simulink model "quadcopter_hover"  (R2022b)
settings: Solver=FixedStepDiscrete  StartTime=0.0  StopTime=40  FixedStep=0.0025  RelTol=1e-3
undefined symbols (not defined in the file or in its folder): f
libraries: instrumentlib x2
settings Model: Creator=HP  LastModifiedBy=HP

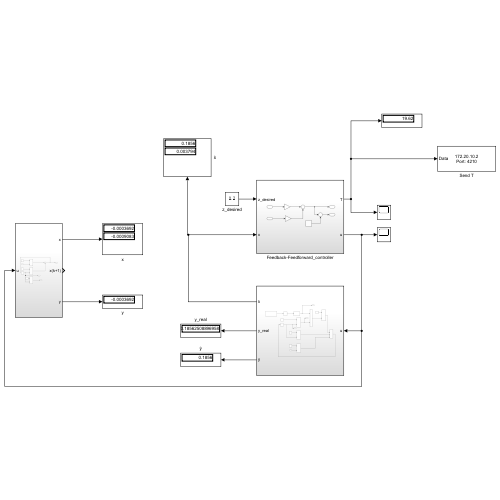
[thumbnail: Simulink's stored preview of the top-level diagram]
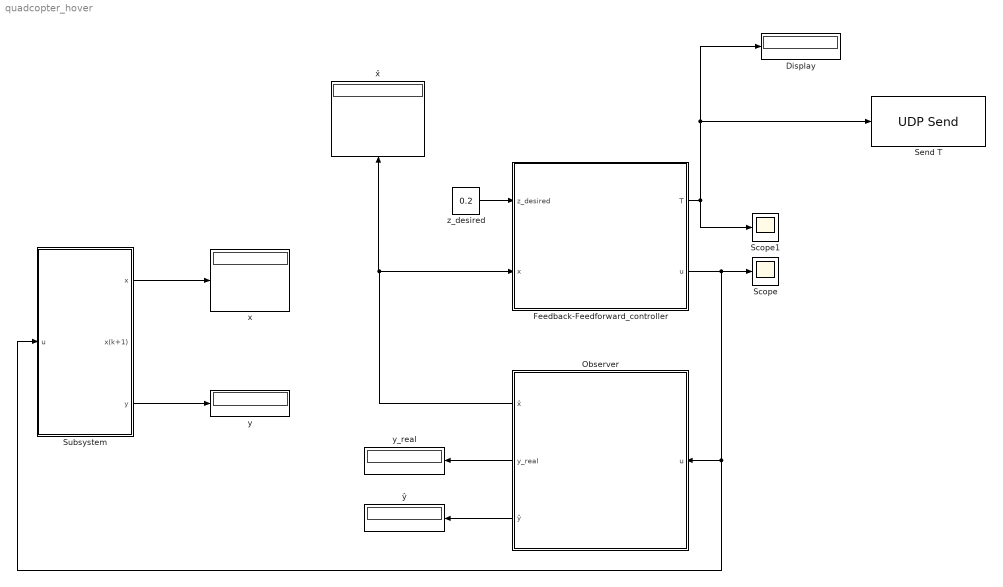
== system quadcopter_hover ==
  Display : Display
  Feedback-Feedforward_controller : Subsystem
  Observer : Subsystem
  Scope : Scope
  Scope1 : Scope
  Send T : instrumentlib/UDP Send  Host=172.20.10.2  Port=4210  LocalAddress=0.0.0.0  LocalPort=4211  EnablePortSharing=off  OutputDatagramPacketSize=512  ByteOrder=big-endian  EnableBlockingMode=on  SimulateUsing=Interpreted execution
  Subsystem : Subsystem
  x : Display
  x̂ : Display
  y : Display
  y_real : Display
  z_desired : Constant  Value=0.2
  ŷ : Display
  wires:
  Feedback-Feedforward_controller/2(u) -> Subsystem/1(u), Observer/1(u), Scope/1
  z_desired/1 -> Feedback-Feedforward_controller/1(z_desired)
  Subsystem/1(x) -> x/1
  Subsystem/3(y) -> y/1
  Observer/1(x̂) -> Feedback-Feedforward_controller/2(x), x̂/1
  Observer/2(y_real) -> y_real/1
  Observer/3(ŷ) -> ŷ/1
  Feedback-Feedforward_controller/1(T) -> Display/1, Send T/1, Scope1/1

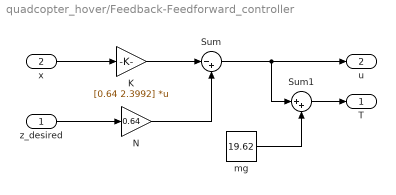
== system quadcopter_hover/Feedback-Feedforward_controller ==
  z_desired : Inport
  x : Inport  Port=2
  K : Gain  Gain=[0.64 2.3992]  Multiplication=Matrix(K*u)
  N : Gain  Gain=0.64
  Sum : Sum  Inputs=|-+
  Sum1 : Sum  Inputs=|++
  mg : Constant  Value=19.62
  T : Outport
  u : Outport  Port=2
  wires:
  x/1 -> K/1
  K/1 -> Sum/1
  z_desired/1 -> N/1
  N/1 -> Sum/2
  Sum/1 -> Sum1/1, u/1
  mg/1 -> Sum1/2
  Sum1/1 -> T/1

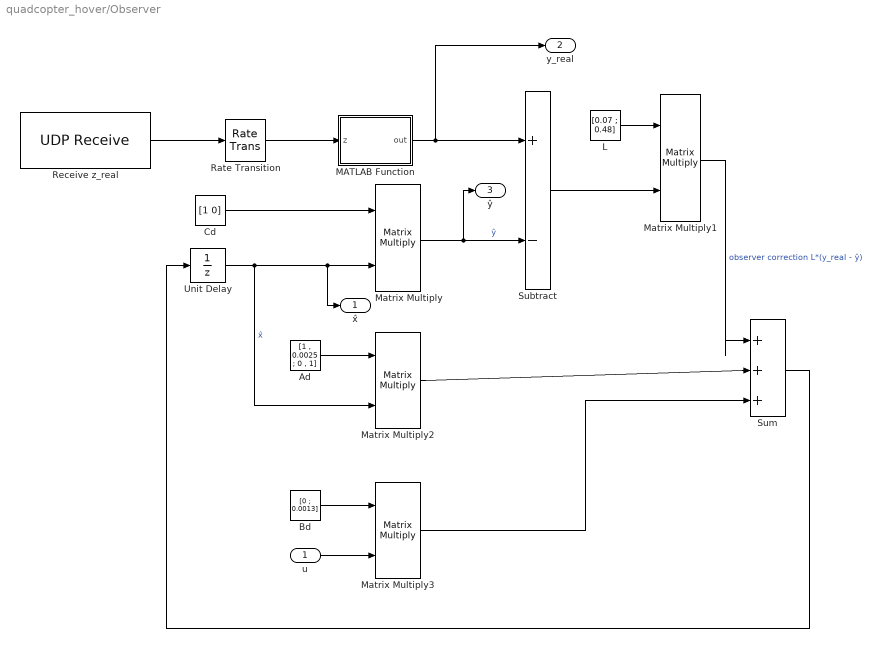
== system quadcopter_hover/Observer ==
  u : Inport
  Ad : Constant  Value=[1 , 0.0025 ; 0 , 1]
  Bd : Constant  Value=[0 ; 0.0013]  VectorParams1D=off
  Cd : Constant  Value=[1 0]  VectorParams1D=off
  L : Constant  Value=[0.07 ; 0.48]
  MATLAB Function : MATLAB Function  TreatAsAtomicUnit=on
  Matrix Multiply{,1..3} (4 alike) : Product  Multiplication=Matrix(*)
  Rate Transition : RateTransition
  Receive z_real : instrumentlib/UDP Receive  LocalAddress=0.0.0.0  LocalPort=5005  EnablePortSharing=off  Host=localhost  Port=5005  GetLatestData=on  DataSize=1  DataType=double  ASCIIFormatting=%f,  Terminator=LF  CustomTerminator=10  ByteOrder=big-endian  EnableBlockingMode=on  Timeout=10  SampleTime=0.01  SimulateUsing=Interpreted execution
  Subtract : Sum  Inputs=+-
  Sum : Sum  Inputs=|+++
  Unit Delay : UnitDelay  InitialCondition=[0 ; 0]  SampleTime=-1  HasFrameUpgradeWarning=on
  x̂ : Outport
  y_real : Outport  Port=2
  ŷ : Outport  Port=3
  wires:
  Cd/1 -> Matrix Multiply/1
  L/1 -> Matrix Multiply1/1
  Subtract/1 -> Matrix Multiply1/2
  Unit Delay/1 -> Matrix Multiply2/2, x̂/1, Matrix Multiply/2  "x̂"
  Matrix Multiply/1 -> ŷ/1, Subtract/2  "ŷ"
  Sum/1 -> Unit Delay/1
  Ad/1 -> Matrix Multiply2/1
  Bd/1 -> Matrix Multiply3/1
  u/1 -> Matrix Multiply3/2
  Matrix Multiply2/1 -> Sum/2
  Matrix Multiply1/1 -> Sum/1  "observer correction L*(y_real - ŷ)"
  Matrix Multiply3/1 -> Sum/3
  Receive z_real/1 -> Rate Transition/1
  MATLAB Function/1(out) -> y_real/1, Subtract/1
  Rate Transition/1 -> MATLAB Function/1(z)

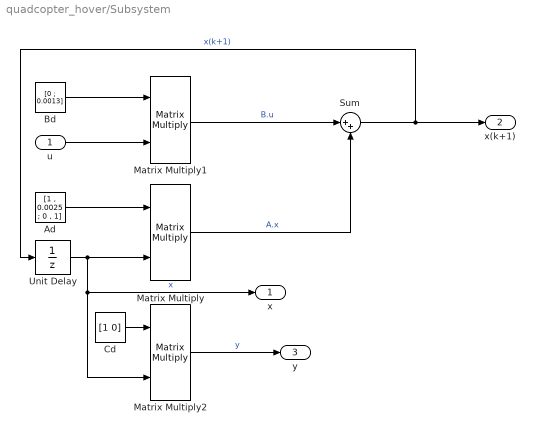
== system quadcopter_hover/Subsystem ==
  u : Inport
  Ad : Constant  Value=[1 , 0.0025 ; 0 , 1]
  Bd : Constant  Value=[0 ; 0.0013]  VectorParams1D=off
  Cd : Constant  Value=[1 0]  VectorParams1D=off
  Matrix Multiply : Product  Multiplication=Matrix(*)
  Matrix Multiply1 : Product  Multiplication=Matrix(*)
  Matrix Multiply2 : Product  Multiplication=Matrix(*)
  Sum : Sum  Inputs=|++
  Unit Delay : UnitDelay  InitialCondition=[0 ; 0]  SampleTime=-1  HasFrameUpgradeWarning=on
  x : Outport
  x(k+1) : Outport  Port=2
  y : Outport  Port=3
  wires:
  Ad/1 -> Matrix Multiply/1
  Unit Delay/1 -> Matrix Multiply/2, x/1, Matrix Multiply2/2  "x"
  Matrix Multiply/1 -> Sum/2  "A.x"
  Bd/1 -> Matrix Multiply1/1
  Matrix Multiply2/1 -> y/1  "y"
  Cd/1 -> Matrix Multiply2/1
  Matrix Multiply1/1 -> Sum/1  "B.u"
  Sum/1 -> x(k+1)/1, Unit Delay/1  "x(k+1)"
  u/1 -> Matrix Multiply1/2

== matlab function quadcopter_hover/Observer/MATLAB Function ==
  data: z input; out output
function out = latchZ(z)
persistent lastZ
if isempty(lastZ)
    lastZ = 0;
end

if isnan(z) || isinf(z)
    out = lastZ;
elseif abs(z - lastZ) > 50  % 💡 sudden jumps? Probably noise
    out = lastZ;
elseif abs(z) < 1e-6
    out = lastZ;
else
    lastZ = z;
    out = z;
end
